simulink model "etude_frequentielle_simple"  (R2016b)
settings: Solver=VariableStepAuto  StartTime=0.0  StopTime=30  MaxStep=0.01  RelTol=1e-3
settings Model: Creator=emiliendurif  LastModifiedBy=emiliendurif

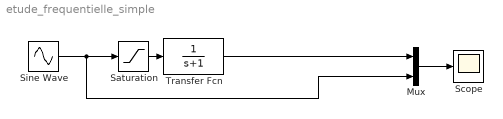
== system etude_frequentielle_simple ==
  Mux : Mux  Inputs=2
  Saturation : Saturate
  Scope : Scope
  Sine Wave : Sin  Amplitude=1.4  SampleTime=0
  Transfer Fcn : TransferFcn  Denominator=[1 1]
  wires:
  Sine Wave/1 -> Mux/2, Saturation/1
  Transfer Fcn/1 -> Mux/1
  Mux/1 -> Scope/1
  Saturation/1 -> Transfer Fcn/1
